simulink library "ddm"  (R2021b)
settings: Solver=VariableStepAuto  StartTime=0.0  StopTime=10.0  RelTol=1e-3
undefined symbols (not defined in the file or in its folder): ADDM_FrTMTqDev_X_Nm, ADDM_RrTMTqDev_X_Nm, ENUM_ADASACCSTA_ERROR, ENUM_ADASACCSTA_OFF, ENUM_ADASACCSTA_STANDBY, ENUM_ALLOWMOV_ALLOWREADY, ENUM_APS, ENUM_BRKSTA_ERROR, ENUM_BRKSTA_OFF, ENUM_BRKSTA_ON, ENUM_BRKSW_INVALID, ENUM_BRKSW_OFF, ENUM_BRKSW_ON, ENUM_CHGPREACTERRSTA_OBCPRE, ENUM_DCDCFAULTSTA_ANYFAULTLV1, ENUM_DCDCFAULTSTA_ANYFAULTLV2, ENUM_DRIVETRAIN_AWD, ENUM_DRIVETRAIN_FWD, ENUM_DRIVETRAIN_RWD, ENUM_EDUDRTSTA_NORMAL, ENUM_EPBSTA_APPLIED, ENUM_EPBSTA_RELEASED, ENUM_GEARACTUALPOSN_INVALID, ENUM_GEARACTUALPOSN_P, ENUM_HVBATTREADYPRE_READY, ENUM_MCUWARN_LV0, ENUM_MCUWARN_LV1, ENUM_MCUWARN_LV2, ENUM_MCUWARN_LV3, ENUM_MCUWARN_NOERROR, ENUM_OBCFAULTSTA_ANYFAULT, ENUM_PAS_R2F2, ENUM_PDFAULT_BATTPDFAIL, ENUM_PDFAULT_DCDCDISABLE, ENUM_PDFAULT_MCUDISABLE, ENUM_PDFAULT_MCUDISCHRG, ENUM_POWERSTA_OFF, ENUM_POWERSTA_ON, ENUM_POWERSTA_READY, ENUM_POWERSTA_STANDBY, ENUM_PRESSINDI_LOW, ENUM_PUFAULT_BATTUPFAIL, ENUM_PUFAULT_DCDCENABLEFAIL, ENUM_PUFAULT_PRECHRGCHKFAIL, ENUM_PUFAULT_SAFETYCHKFAIL, ENUM_PUSTATE_COMPLETED, ENUM_PWRSTASW_OFF, ENUM_PWRSTASW_OFFA, ENUM_PWRSTASW_OFFCHVCHRG, ENUM_PWRSTASW_OFFCLVCHRG, ENUM_PWRSTASW_ON, ENUM_PWRSTASW_ONHVCHRG, ENUM_PWRSTASW_READY, ENUM_PWRSTASW_STANDBY, ENUM_SHIFTCOMMAND_P, ENUM_SHIFTERERRSTA_PBUTTONFAILURE, ENUM_VEHMALFUNLV_2ND, ENUM_VEHMALFUNLV_3RD, ENUM_VEHMALFUNLV_4TH, ENUM_VEHMALFUNLV_NORMAL ... (+459)
libraries: hcu_lib x521, $bdroot x5, simulink x3
(part 22 of 25)

== system ddm/DDM/DDM/PMM/power up and power down/MCU active discharge fail ==
  note: Test Pass Criteria
  note: Test Detection Criteria
  note: Release Condition After Decision
  note: Diagnostics and Fault Handling
  task_time_s : Inport
  VPMM_PowerSta_enum : Inport  Port=2
  VPMM_PwrStaSW_enum : Inport  Port=3
  VPMM_PowerDownFault_enum : Inport  Port=4
  DTC_clear_request : Inport  Port=5
  VPMM_MCUDCBusMaxVolt_V : Inport  Port=6
  Constant : Constant  Value=ENUM_PDFAULT_MCUDISCHRG
  Constant1 : Constant  Value=FALSE
  Constant12 : Constant  Value=ENUM_PWRSTASW_OFF
  Constant13 : Constant  Value=FALSE
  Constant14 : Constant  Value=ZERO_INT
  Constant18 : Constant  Value=KPMM_MCUDischrgVolt_V
  Constant19 : Constant  Value=KDDM_MCUActDTC_cnt
  Constant2 : Constant  Value=TRUE
  Constant26 : Constant  Value=KDDM_MCUActDTC_cnt
  Constant29 : Constant  Value=FALSE
  Constant3 : Constant  Value=KDDM_PwrUpDnDiagnosisOffSW_flg
  Constant4 : Constant  Value=ENUM_POWERSTA_OFF
  Constant41 : Constant  Value=KDDM_MCUActDetTO_s
  Constant5 : Constant  Value=ENUM_PWRSTASW_OFF
  Constant6 : Constant  Value=TRUE
  Constant7 : Constant  Value=KDDM_MCUActPassTO_s
  Constant8 : Constant  Value=KDDM_MCUActPassTO_s
  Constant9 : Constant  Value=ENUM_POWERSTA_STANDBY
  DTC_Couter1 : hcu_lib/Basic_Blocks/DTC_Couter
  DTC_Info : hcu_lib/Basic_Blocks/DTC_Info
  Equal1 : RelationalOperator  Operator===  OutDataTypeStr=boolean  RndMeth=Simplest
  Equal11 : RelationalOperator  Operator=<=  OutDataTypeStr=boolean  RndMeth=Simplest
  Equal3 : RelationalOperator  Operator===  OutDataTypeStr=boolean  RndMeth=Simplest
  Equal5 : RelationalOperator  Operator=~=  OutDataTypeStr=boolean  RndMeth=Simplest
  Equal7 : RelationalOperator  Operator=~=  OutDataTypeStr=boolean  RndMeth=Simplest
  Equal8 : RelationalOperator  OutDataTypeStr=boolean  RndMeth=Simplest
  Equal9 : RelationalOperator  Operator===  OutDataTypeStr=boolean  RndMeth=Simplest
  Logical Operator13 : Logic  Operator=NOT  AllPortsSameDT=off  OutDataTypeStr=boolean
  Logical Operator14 : Logic  Operator=OR  Inputs=5  AllPortsSameDT=off  OutDataTypeStr=boolean
  Logical Operator16 : Logic  AllPortsSameDT=off  OutDataTypeStr=boolean
  Relational Operator1 : RelationalOperator  Operator=>  OutDataTypeStr=boolean  RndMeth=Simplest
  Switch{1..3,6} (4 alike) : Switch  Criteria=u2 ~= 0
  Terminator : Terminator
  Test Detection Criteria1 : hcu_lib/Basic_Blocks/Test Detection Criteria
  Timer2 : hcu_lib/Basic_Blocks/Timer
  Unit Delay1 : UnitDelay  SampleTime=-1  HasFrameUpgradeWarning=on
  VDDM_MCUActDTC_raw32 : Outport
  VDDM_MCUActDisFail_flg : Outport  Port=2
  VDDM_MCUActCFS_flg : Outport  Port=3
  wires:
  Switch1/1 -> VDDM_MCUActDisFail_flg/1  "VDDM_MCUActDisFail_flg"
  [VDDM_MCUActCFS_flg] -> Switch1/2, VDDM_MCUActCFS_flg/1
  Constant1/1 -> Switch1/3
  Constant2/1 -> Switch1/1
  [VDDM_MCUActPass_flg] -> Logical Operator14/3
  Constant18/1 -> Equal11/2
  Equal11/1 -> Logical Operator14/4
  [VPMM_MCUDCBusMaxVolt_V] -> Equal11/1
  Test Detection Criteria1/1 -> [VDDM_MCUActDet_flg]  "VDDM_MCUActDet_flg"
  Constant12/1 -> Equal7/2
  Relational Operator1/1 -> Terminator/1  "VDDM_MCUActDFS_flg"
  Constant7/1 -> Timer2/4
  Constant41/1 -> Test Detection Criteria1/4
  Logical Operator16/1 -> Logical Operator14/1
  [VPMM_PowerSta_enum] -> Unit Delay1/1
  [VPMM_PwrStaSW_enum] -> Equal7/1
  Timer2/1 -> Equal8/1
  DTC_Couter1/2 -> Relational Operator1/1  "VDDM_MCUActDTC_cnt"
  Constant4/1 -> Equal9/2
  [DTC_clear_request] -> Logical Operator14/2
  [VDDM_MCUActCFSRls_flg] -> DTC_Couter1/2
  [VPMM_PowerSta_enum] -> Equal3/1
  Unit Delay1/1 -> Equal9/1
  Constant9/1 -> Equal3/2
  Switch3/1 -> Switch6/3
  Logical Operator13/1 -> Timer2/1
  [VDDM_MCUActChk_flg] -> Switch3/1
  [task_time_s] -> Timer2/3
  Equal9/1 -> Logical Operator16/1
  Constant3/1 -> Logical Operator14/5
  Constant19/1 -> DTC_Couter1/3
  Switch2/1 -> Logical Operator13/1, Timer2/2
  Constant29/1 -> Switch6/1
  [task_time_s] -> Test Detection Criteria1/2
  Switch6/1 -> Test Detection Criteria1/1
  Constant5/1 -> Equal5/2
  Equal3/1 -> Logical Operator16/2
  Constant14/1 -> Relational Operator1/2
  Constant13/1 -> Switch3/3
  Constant8/1 -> Equal8/2
  Logical Operator14/1 -> [VDDM_MCUActCFSRls_flg]  "VDDM_MCUActCFSRls_flg"
  Constant26/1 -> Test Detection Criteria1/3
  [VDDM_MCUActDet_flg] -> DTC_Couter1/1
  Equal7/1 -> Switch3/2
  Constant6/1 -> Switch2/3
  [VDDM_MCUActCFSRls_flg] -> Switch6/2
  Equal8/1 -> [VDDM_MCUActPass_flg]  "VDDM_MCUActPass_flg"
  [VDDM_MCUActChk_flg] -> Switch2/1
  [VPMM_PwrStaSW_enum] -> Equal5/1
  Equal5/1 -> Switch2/2
  DTC_Couter1/1 -> [VDDM_MCUActCFS_flg]  "VDDM_MCUActCFS_flg"
  VPMM_PowerSta_enum/1 -> [VPMM_PowerSta_enum]
  VPMM_PwrStaSW_enum/1 -> [VPMM_PwrStaSW_enum]
  task_time_s/1 -> [task_time_s]
  DTC_clear_request/1 -> [DTC_clear_request]
  Constant/1 -> Equal1/2
  VPMM_PowerDownFault_enum/1 -> Equal1/1
  Equal1/1 -> [VDDM_MCUActChk_flg]
  DTC_Info/1 -> VDDM_MCUActDTC_raw32/1  "VDDM_MCUActDTC_raw32"
  [VDDM_MCUActPass_flg] -> DTC_Info/2
  [VDDM_MCUActCFS_flg] -> DTC_Info/3
  [VDDM_MCUActDet_flg] -> DTC_Info/1
  [DTC_clear_request] -> DTC_Info/4
  VPMM_MCUDCBusMaxVolt_V/1 -> [VPMM_MCUDCBusMaxVolt_V]

== system ddm/DDM/DDM/PMM/power up and power down/MCU disable fail ==
  note: Test Detection Criteria
  note: Test Pass Criteria
  note: Diagnostics and Fault Handling
  note: Release Condition After Decision
  task_time_s : Inport
  VPMM_PowerSta_enum : Inport  Port=2
  VPMM_PwrStaSW_enum : Inport  Port=3
  VPMM_PowerDownFault_enum : Inport  Port=4
  DTC_clear_request : Inport  Port=5
  Constant : Constant  Value=ENUM_PDFAULT_MCUDISABLE
  Constant1 : Constant  Value=KDDM_PwrUpDnDiagnosisOffSW_flg
  Constant12 : Constant  Value=ENUM_PWRSTASW_OFF
  Constant13 : Constant  Value=FALSE
  Constant14 : Constant  Value=ZERO_INT
  Constant18 : Constant  Value=KDDM_MCUDisDTC_cnt
  Constant2 : Constant  Value=ENUM_PWRSTASW_OFF
  Constant23 : Constant  Value=TRUE
  Constant26 : Constant  Value=KDDM_MCUDisDTC_cnt
  Constant29 : Constant  Value=FALSE
  Constant3 : Constant  Value=ENUM_POWERSTA_OFF
  Constant4 : Constant  Value=KDDM_MCUDisPassTO_s
  Constant41 : Constant  Value=KDDM_MCUDisDetTO_s
  Constant8 : Constant  Value=ENUM_POWERSTA_STANDBY
  Constant9 : Constant  Value=KDDM_MCUDisPassTO_s
  DTC_Couter1 : hcu_lib/Basic_Blocks/DTC_Couter
  DTC_Info : hcu_lib/Basic_Blocks/DTC_Info
  Equal1 : RelationalOperator  Operator===  OutDataTypeStr=boolean  RndMeth=Simplest
  Equal10 : RelationalOperator  Operator===  OutDataTypeStr=boolean  RndMeth=Simplest
  Equal2 : RelationalOperator  Operator=~=  OutDataTypeStr=boolean  RndMeth=Simplest
  Equal5 : RelationalOperator  Operator=~=  OutDataTypeStr=boolean  RndMeth=Simplest
  Equal8 : RelationalOperator  OutDataTypeStr=boolean  RndMeth=Simplest
  Equal9 : RelationalOperator  Operator===  OutDataTypeStr=boolean  RndMeth=Simplest
  Logical Operator13 : Logic  Operator=NOT  AllPortsSameDT=off  OutDataTypeStr=boolean
  Logical Operator14 : Logic  Operator=OR  Inputs=4  AllPortsSameDT=off  OutDataTypeStr=boolean
  Logical Operator16 : Logic  AllPortsSameDT=off  OutDataTypeStr=boolean
  Relational Operator1 : RelationalOperator  Operator=>  OutDataTypeStr=boolean  RndMeth=Simplest
  Switch1 : Switch  Criteria=u2 ~= 0
  Switch3 : Switch  Criteria=u2 ~= 0
  Switch6 : Switch  Criteria=u2 ~= 0
  Terminator : Terminator
  Test Detection Criteria1 : hcu_lib/Basic_Blocks/Test Detection Criteria
  Timer2 : hcu_lib/Basic_Blocks/Timer
  Unit Delay1 : UnitDelay  SampleTime=-1  HasFrameUpgradeWarning=on
  VDDM_MCUDisDTC_raw32 : Outport
  VDDM_MCUDisCFS_flg : Outport  Port=2
  wires:
  [VDDM_MCUDisCFS_flg] -> VDDM_MCUDisCFS_flg/1
  Constant23/1 -> Switch1/3
  [VDDM_MCUDisChk_flg] -> Switch1/1
  Equal2/1 -> Switch1/2
  Constant2/1 -> Equal2/2
  [VPMM_PwrStaSW_enum] -> Equal2/1
  DTC_Couter1/1 -> [VDDM_MCUDisCFS_flg]  "VDDM_MCUDisCFS_flg"
  [VPMM_PwrStaSW_enum] -> Equal5/1
  Equal8/1 -> [VDDM_MCUDisPass_flg]  "VDDM_MCUDisPass_flg"
  [task_time_s] -> Test Detection Criteria1/2
  Constant26/1 -> Test Detection Criteria1/3
  Unit Delay1/1 -> Equal9/1
  [VDDM_MCUDisChk_flg] -> Switch3/1
  Test Detection Criteria1/1 -> [VDDM_MCUDisDet_flg]  "VDDM_MCUDisDet_flg"
  Equal10/1 -> Logical Operator16/2
  DTC_Couter1/2 -> Relational Operator1/1  "VDDM_MCUDisDTC_cnt"
  Switch6/1 -> Test Detection Criteria1/1
  Constant4/1 -> Timer2/4
  Switch1/1 -> Logical Operator13/1, Timer2/2
  Logical Operator14/1 -> [VDDM_MCUDisCFSRls_flg]  "VDDM_MCUDisCFSRls_flg"
  Switch3/1 -> Switch6/3
  Constant13/1 -> Switch3/3
  Constant14/1 -> Relational Operator1/2
  [VDDM_MCUDisPass_flg] -> Logical Operator14/3
  [DTC_clear_request] -> Logical Operator14/2
  Constant29/1 -> Switch6/1
  Equal5/1 -> Switch3/2
  Constant9/1 -> Equal8/2
  [VDDM_MCUDisCFSRls_flg] -> DTC_Couter1/2
  Constant41/1 -> Test Detection Criteria1/4
  Logical Operator16/1 -> Logical Operator14/1
  Constant12/1 -> Equal5/2
  Logical Operator13/1 -> Timer2/1
  Equal9/1 -> Logical Operator16/1
  Timer2/1 -> Equal8/1
  Constant18/1 -> DTC_Couter1/3
  Constant1/1 -> Logical Operator14/4
  [VPMM_PowerSta_enum] -> Unit Delay1/1
  [VPMM_PowerSta_enum] -> Equal10/1
  Constant3/1 -> Equal9/2
  Constant8/1 -> Equal10/2
  [task_time_s] -> Timer2/3
  [VDDM_MCUDisDet_flg] -> DTC_Couter1/1
  Relational Operator1/1 -> Terminator/1  "VDDM_MCUDisDFS_flg"
  [VDDM_MCUDisCFSRls_flg] -> Switch6/2
  task_time_s/1 -> [task_time_s]
  VPMM_PwrStaSW_enum/1 -> [VPMM_PwrStaSW_enum]
  VPMM_PowerSta_enum/1 -> [VPMM_PowerSta_enum]
  Constant/1 -> Equal1/2
  VPMM_PowerDownFault_enum/1 -> Equal1/1
  DTC_clear_request/1 -> [DTC_clear_request]
  Equal1/1 -> [VDDM_MCUDisChk_flg]
  DTC_Info/1 -> VDDM_MCUDisDTC_raw32/1  "VDDM_MCUDisDTC_raw32"
  [VDDM_MCUDisPass_flg] -> DTC_Info/2
  [VDDM_MCUDisCFS_flg] -> DTC_Info/3
  [VDDM_MCUDisDet_flg] -> DTC_Info/1
  [DTC_clear_request] -> DTC_Info/4

== system ddm/DDM/DDM/PMM/power up and power down/MCU ready for precharge fail ==
  note: Diagnostics and Fault Handling
  note: Test Detection Criteria
  note: Test Pass Criteria
  note: Release Condition After Decision
  task_time_s : Inport
  VPMM_PowerSta_enum : Inport  Port=2
  VPMM_PwrStaSW_enum : Inport  Port=3
  VPMM_MCUReady4Pre_flg : Inport  Port=4
  VPMM_PowerUpFault_enum : Inport  Port=5
  DTC_clear_request : Inport  Port=6
  VPMM_PowerUpState_enum : Inport  Port=7
  Constant : Constant  Value=ENUM_PUFAULT_PRECHRGCHKFAIL
  Constant12 : Constant  Value=ENUM_PWRSTASW_OFF
  Constant13 : Constant  Value=FALSE
  Constant14 : Constant  Value=ZERO_INT
  Constant17 : Constant  Value=KDDM_PwrUpDnDiagnosisOffSW_flg
  Constant18 : Constant  Value=KDDM_MCU4PrePassTO_s
  Constant22 : Constant  Value=ENUM_POWERSTA_OFF
  Constant28 : Constant  Value=KDDM_MCU4PrePassTO_s
  Constant29 : Constant  Value=FALSE
  Constant3 : Constant  Value=KDDM_MCU4PreDTC_cnt
  Constant4 : Constant  Value=FALSE
  Constant41 : Constant  Value=KDDM_MCU4PreDetTO_s
  Constant5 : Constant  Value=ENUM_PUSTATE_COMPLETED
  Constant6 : Constant  Value=TRUE
  Constant7 : Constant  Value=ENUM_POWERSTA_STANDBY
  Constant9 : Constant  Value=KDDM_MCU4PreDTC_cnt
  DTC_Couter1 : hcu_lib/Basic_Blocks/DTC_Couter
  DTC_Info : hcu_lib/Basic_Blocks/DTC_Info
  Equal{1,3,8..9} (4 alike) : RelationalOperator  Operator===  OutDataTypeStr=boolean  RndMeth=Simplest
  Equal4 : RelationalOperator  Operator=~=  OutDataTypeStr=boolean  RndMeth=Simplest
  Equal7 : RelationalOperator  OutDataTypeStr=boolean  RndMeth=Simplest
  Logical Operator13 : Logic  Operator=NOT  AllPortsSameDT=off  OutDataTypeStr=boolean
  Logical Operator14 : Logic  Operator=OR  Inputs=4  AllPortsSameDT=off  OutDataTypeStr=boolean
  Logical Operator16 : Logic  AllPortsSameDT=off  OutDataTypeStr=boolean
  Logical Operator4 : Logic  AllPortsSameDT=off  OutDataTypeStr=boolean
  Logical Operator5 : Logic  Operator=NOT  AllPortsSameDT=off  OutDataTypeStr=boolean
  Relational Operator1 : RelationalOperator  Operator=>  OutDataTypeStr=boolean  RndMeth=Simplest
  Switch1 : Switch  Criteria=u2 ~= 0
  Switch3 : Switch  Criteria=u2 ~= 0
  Switch6 : Switch  Criteria=u2 ~= 0
  Terminator : Terminator
  Test Detection Criteria1 : hcu_lib/Basic_Blocks/Test Detection Criteria
  Timer2 : hcu_lib/Basic_Blocks/Timer
  Unit Delay1 : UnitDelay  SampleTime=-1  HasFrameUpgradeWarning=on
  VDDM_MCU4PreDTC_raw32 : Outport
  VDDM_MCU4PreCFS_flg : Outport  Port=2
  wires:
  [VDDM_MCU4PreCFS_flg] -> VDDM_MCU4PreCFS_flg/1
  Constant9/1 -> Test Detection Criteria1/3
  [VDDM_MCU4PreCFSRls_flg] -> DTC_Couter1/2
  Test Detection Criteria1/1 -> [VDDM_MCU4PreDet_flg]  "VDDM_MCU4PreDet_flg"
  Logical Operator14/1 -> [VDDM_MCU4PreCFSRls_flg]  "VDDM_MCU4PreCFSRls_flg"
  Constant4/1 -> Switch1/1
  Switch1/1 -> Logical Operator13/1, Timer2/2
  [DTC_clear_request] -> Logical Operator14/2
  [VPMM_PowerSta_enum] -> Unit Delay1/1
  Constant14/1 -> Relational Operator1/2
  Equal3/1 -> Switch1/2
  Equal4/1 -> Switch3/2
  Switch3/1 -> Switch6/3
  [VPMM_PowerSta_enum] -> Equal9/1
  [VDDM_MCU4PrePass_flg] -> Logical Operator14/3
  Constant7/1 -> Equal9/2
  Constant5/1 -> Equal3/2
  Constant29/1 -> Switch6/1
  Unit Delay1/1 -> Equal8/1
  Constant12/1 -> Equal4/2
  Constant17/1 -> Logical Operator14/4
  [task_time_s] -> Test Detection Criteria1/2
  [VDDM_MCU4PreCFSRls_flg] -> Switch6/2
  [VDDM_MCU4PreDet_flg] -> DTC_Couter1/1
  Constant22/1 -> Equal8/2
  Constant13/1 -> Switch3/3
  Constant3/1 -> DTC_Couter1/3
  Switch6/1 -> Test Detection Criteria1/1
  Equal9/1 -> Logical Operator16/2
  Logical Operator13/1 -> Timer2/1
  DTC_Couter1/2 -> Relational Operator1/1  "VDDM_MCU4PreDTC_cnt"
  Constant6/1 -> Switch1/3
  Constant41/1 -> Test Detection Criteria1/4
  [task_time_s] -> Timer2/3
  [VPMM_PowerUpState_enum] -> Equal3/1
  Equal8/1 -> Logical Operator16/1
  Timer2/1 -> Equal7/1
  Logical Operator16/1 -> Logical Operator14/1
  Equal7/1 -> [VDDM_MCU4PrePass_flg]  "VDDM_MCU4PrePass_flg"
  [VPMM_PwrStaSW_enum] -> Equal4/1
  [VDDM_MCU4PreChk_flg] -> Switch3/1
  Relational Operator1/1 -> Terminator/1  "VDDM_MCU4PreDFS_flg"
  Constant28/1 -> Equal7/2
  DTC_Couter1/1 -> [VDDM_MCU4PreCFS_flg]  "VDDM_MCU4PreCFS_flg"
  Constant18/1 -> Timer2/4
  task_time_s/1 -> [task_time_s]
  VPMM_PwrStaSW_enum/1 -> [VPMM_PwrStaSW_enum]
  VPMM_PowerSta_enum/1 -> [VPMM_PowerSta_enum]
  DTC_clear_request/1 -> [DTC_clear_request]
  Constant/1 -> Equal1/2
  VPMM_PowerUpFault_enum/1 -> Equal1/1
  Logical Operator5/1 -> Logical Operator4/1
  Equal1/1 -> Logical Operator4/2
  Logical Operator4/1 -> [VDDM_MCU4PreChk_flg]
  VPMM_MCUReady4Pre_flg/1 -> Logical Operator5/1
  [VDDM_MCU4PrePass_flg] -> DTC_Info/2
  DTC_Info/1 -> VDDM_MCU4PreDTC_raw32/1  "VDDM_MCU4PreDTC_raw32"
  [VDDM_MCU4PreCFS_flg] -> DTC_Info/3
  [VDDM_MCU4PreDet_flg] -> DTC_Info/1
  [DTC_clear_request] -> DTC_Info/4
  VPMM_PowerUpState_enum/1 -> [VPMM_PowerUpState_enum]

== system ddm/DDM/DDM/PMM/power up and power down/Mid level system safety check fail ==
  note: Release Condition After Decision
  note: Diagnostics and Fault Handling
  note: Test Detection Criteria
  note: Test Pass Criteria
  task_time_s : Inport
  VPMM_PowerSta_enum : Inport  Port=2
  VPMM_PwrStaSW_enum : Inport  Port=3
  VDDM_MidLvSaChkChk_flg : Inport  Port=4
  VPMM_PowerUpFault_enum : Inport  Port=5
  DTC_clear_request : Inport  Port=6
  VPMM_PowerUpState_enum : Inport  Port=7
  Constant : Constant  Value=ENUM_PUFAULT_SAFETYCHKFAIL
  Constant12 : Constant  Value=ENUM_PWRSTASW_OFF
  Constant13 : Constant  Value=FALSE
  Constant14 : Constant  Value=ZERO_INT
  Constant17 : Constant  Value=KDDM_PwrUpDnDiagnosisOffSW_flg
  Constant18 : Constant  Value=KDDM_MidLvSaChkDTC_cnt
  Constant22 : Constant  Value=ENUM_POWERSTA_OFF
  Constant28 : Constant  Value=KDDM_MidLvSaChkPassTO_s
  Constant29 : Constant  Value=FALSE
  Constant3 : Constant  Value=KDDM_MidLvSaChkDTC_cnt
  Constant30 : Constant  Value=KDDM_MidLvSaChkPassTO_s
  Constant4 : Constant  Value=FALSE
  Constant41 : Constant  Value=KDDM_MidLvSaChkDetTO_s
  Constant5 : Constant  Value=ENUM_PUSTATE_COMPLETED
  Constant6 : Constant  Value=TRUE
  Constant7 : Constant  Value=ENUM_POWERSTA_STANDBY
  DTC_Couter1 : hcu_lib/Basic_Blocks/DTC_Couter
  DTC_Info : hcu_lib/Basic_Blocks/DTC_Info
  Equal{1,3,8..9} (4 alike) : RelationalOperator  Operator===  OutDataTypeStr=boolean  RndMeth=Simplest
  Equal4 : RelationalOperator  Operator=~=  OutDataTypeStr=boolean  RndMeth=Simplest
  Equal7 : RelationalOperator  OutDataTypeStr=boolean  RndMeth=Simplest
  Logical Operator13 : Logic  Operator=NOT  AllPortsSameDT=off  OutDataTypeStr=boolean
  Logical Operator14 : Logic  Operator=OR  Inputs=4  AllPortsSameDT=off  OutDataTypeStr=boolean
  Logical Operator16 : Logic  AllPortsSameDT=off  OutDataTypeStr=boolean
  Logical Operator4 : Logic  Operator=NOT  AllPortsSameDT=off  OutDataTypeStr=boolean
  Logical Operator5 : Logic  AllPortsSameDT=off  OutDataTypeStr=boolean
  Relational Operator1 : RelationalOperator  Operator=>  OutDataTypeStr=boolean  RndMeth=Simplest
  Switch1 : Switch  Criteria=u2 ~= 0
  Switch3 : Switch  Criteria=u2 ~= 0
  Switch6 : Switch  Criteria=u2 ~= 0
  Terminator : Terminator
  Test Detection Criteria1 : hcu_lib/Basic_Blocks/Test Detection Criteria
  Timer2 : hcu_lib/Basic_Blocks/Timer
  Unit Delay1 : UnitDelay  SampleTime=-1  HasFrameUpgradeWarning=on
  VDDM_MidLvSaChkDTC_raw32 : Outport
  VDDM_MidLvSaChkCFS_flg : Outport  Port=2
  wires:
  [VDDM_MidLvSaChkCFS_flg] -> VDDM_MidLvSaChkCFS_flg/1
  Equal4/1 -> Switch3/2
  Relational Operator1/1 -> Terminator/1  "VDDM_MidLvSaChkDFS_flg"
  [DTC_clear_request] -> Logical Operator14/2
  Constant29/1 -> Switch6/1
  Logical Operator14/1 -> [VDDM_MidLvSaChkCFSRls_flg]  "VDDM_MidLvSaChkCFSRls_flg"
  [VDDM_MidLvSaChkPass_flg] -> Logical Operator14/3
  Constant6/1 -> Switch1/3
  [task_time_s] -> Test Detection Criteria1/2
  Constant14/1 -> Relational Operator1/2
  Constant13/1 -> Switch3/3
  DTC_Couter1/1 -> [VDDM_MidLvSaChkCFS_flg]  "VDDM_MidLvSaChkCFS_flg"
  Equal7/1 -> [VDDM_MidLvSaChkPass_flg]  "VDDM_MidLvSaChkPass_flg"
  Switch1/1 -> Logical Operator13/1, Timer2/2
  Switch3/1 -> Switch6/3
  Constant28/1 -> Timer2/4
  Constant5/1 -> Equal3/2
  [VPMM_PwrStaSW_enum] -> Equal4/1
  Equal9/1 -> Logical Operator16/2
  Constant30/1 -> Equal7/2
  Constant3/1 -> Test Detection Criteria1/3
  DTC_Couter1/2 -> Relational Operator1/1  "VDDM_MidLvSaChkDTC_cnt"
  Constant4/1 -> Switch1/1
  [VPMM_PowerUpState_enum] -> Equal3/1
  Unit Delay1/1 -> Equal8/1
  Constant7/1 -> Equal9/2
  [task_time_s] -> Timer2/3
  Constant22/1 -> Equal8/2
  [VPMM_PowerSta_enum] -> Equal9/1
  Constant17/1 -> Logical Operator14/4
  Switch6/1 -> Test Detection Criteria1/1
  [VPMM_PowerSta_enum] -> Unit Delay1/1
  Logical Operator13/1 -> Timer2/1
  [VDDM_MidLvSaChkChk_flg] -> Switch3/1
  Timer2/1 -> Equal7/1
  Constant12/1 -> Equal4/2
  Equal8/1 -> Logical Operator16/1
  Equal3/1 -> Switch1/2
  Constant41/1 -> Test Detection Criteria1/4
  Logical Operator16/1 -> Logical Operator14/1
  Test Detection Criteria1/1 -> [VDDM_MidLvSaChkDet_flg]  "VDDM_MidLvSaChkDet_flg"
  [VDDM_MidLvSaChkCFSRls_flg] -> DTC_Couter1/2
  [VDDM_MidLvSaChkDet_flg] -> DTC_Couter1/1
  [VDDM_MidLvSaChkCFSRls_flg] -> Switch6/2
  Constant18/1 -> DTC_Couter1/3
  VPMM_PowerSta_enum/1 -> [VPMM_PowerSta_enum]
  VPMM_PwrStaSW_enum/1 -> [VPMM_PwrStaSW_enum]
  task_time_s/1 -> [task_time_s]
  Constant/1 -> Equal1/2
  Equal1/1 -> Logical Operator5/2
  Logical Operator4/1 -> Logical Operator5/1
  VPMM_PowerUpFault_enum/1 -> Equal1/1
  Logical Operator5/1 -> [VDDM_MidLvSaChkChk_flg]
  VDDM_MidLvSaChkChk_flg/1 -> Logical Operator4/1
  DTC_clear_request/1 -> [DTC_clear_request]
  DTC_Info/1 -> VDDM_MidLvSaChkDTC_raw32/1  "VDDM_MidLvSaChkDTC_raw32"
  [VDDM_MidLvSaChkPass_flg] -> DTC_Info/2
  [VDDM_MidLvSaChkCFS_flg] -> DTC_Info/3
  [VDDM_MidLvSaChkDet_flg] -> DTC_Info/1
  [DTC_clear_request] -> DTC_Info/4
  VPMM_PowerUpState_enum/1 -> [VPMM_PowerUpState_enum]

== system ddm/DDM/DDM/PMM/power up and power down/OBC ready for precharge fail ==
  note: Release Condition After Decision
  note: Test Detection Criteria
  note: Diagnostics and Fault Handling
  note: Test Pass Criteria
  task_time_s : Inport
  VPMM_PowerSta_enum : Inport  Port=2
  VPMM_PwrStaSW_enum : Inport  Port=3
  VPMM_HVChrgPreActionErrSta_enum : Inport  Port=4
  DTC_clear_request : Inport  Port=5
  Constant12 : Constant  Value=ENUM_PWRSTASW_OFFCLVCHRG
  Constant13 : Constant  Value=ENUM_PWRSTASW_ONHVCHRG
  Constant14 : Constant  Value=ZERO_INT
  Constant22 : Constant  Value=ENUM_PWRSTASW_ON
  Constant28 : Constant  Value=FALSE
  Constant29 : Constant  Value=ENUM_PWRSTASW_OFFCHVCHRG
  Constant3 : Constant  Value=ENUM_CHGPREACTERRSTA_OBCPRE
  Constant30 : Constant  Value=KDDM_OBC4PreDetTO_s
  Constant31 : Constant  Value=FALSE
  Constant32 : Constant  Value=ENUM_POWERSTA_OFF
  Constant33 : Constant  Value=KDDM_OBC4PreDTC_cnt
  Constant34 : Constant  Value=ENUM_POWERSTA_STANDBY
  Constant35 : Constant  Value=ENUM_PWRSTASW_OFFCLVCHRG
  Constant36 : Constant  Value=TRUE
  Constant37 : Constant  Value=ENUM_PWRSTASW_ONHVCHRG
  Constant39 : Constant  Value=ENUM_PWRSTASW_ON
  Constant41 : Constant  Value=ENUM_PWRSTASW_OFFCHVCHRG
  Constant42 : Constant  Value=KDDM_OBC4PrePassTO_s
  Constant45 : Constant  Value=KDDM_OBC4PrePassTO_s
  Constant46 : Constant  Value=KDDM_OBC4PreDTC_cnt
  Constant9 : Constant  Value=KDDM_PwrUpDnDiagnosisOffSW_flg
  DTC_Couter1 : hcu_lib/Basic_Blocks/DTC_Couter
  DTC_Info : hcu_lib/Basic_Blocks/DTC_Info
  Equal{10..12,14..20,24} (11 alike) : RelationalOperator  Operator===  OutDataTypeStr=boolean  RndMeth=Simplest
  Equal13 : RelationalOperator  OutDataTypeStr=boolean  RndMeth=Simplest
  Logical Operator10 : Logic  Operator=OR  Inputs=4  AllPortsSameDT=off  OutDataTypeStr=boolean
  Logical Operator13 : Logic  Operator=NOT  AllPortsSameDT=off  OutDataTypeStr=boolean
  Logical Operator14 : Logic  Operator=OR  Inputs=4  AllPortsSameDT=off  OutDataTypeStr=boolean
  Logical Operator16 : Logic  AllPortsSameDT=off  OutDataTypeStr=boolean
  Logical Operator9 : Logic  Operator=OR  Inputs=4  AllPortsSameDT=off  OutDataTypeStr=boolean
  Relational Operator1 : RelationalOperator  Operator=>  OutDataTypeStr=boolean  RndMeth=Simplest
  Switch3 : Switch  Criteria=u2 ~= 0
  Switch6 : Switch  Criteria=u2 ~= 0
  Switch7 : Switch  Criteria=u2 ~= 0
  Terminator : Terminator
  Test Detection Criteria1 : hcu_lib/Basic_Blocks/Test Detection Criteria
  Timer2 : hcu_lib/Basic_Blocks/Timer
  Unit Delay1 : UnitDelay  SampleTime=-1  HasFrameUpgradeWarning=on
  VDDM_OBC4PreDTC_raw32 : Outport
  VDDM_OBC4PreCFS_flg : Outport  Port=2
  wires:
  [VDDM_OBC4PreCFS_flg] -> VDDM_OBC4PreCFS_flg/1
  Constant39/1 -> Equal17/2
  [VPMM_PwrStaSW_enum] -> Equal17/1
  Equal19/1 -> Logical Operator10/1
  [VPMM_PwrStaSW_enum] -> Equal19/1
  [VPMM_PwrStaSW_enum] -> Equal20/1
  Constant41/1 -> Equal19/2
  Equal20/1 -> Logical Operator10/4
  Constant37/1 -> Equal20/2
  Constant36/1 -> Switch6/3
  [VDDM_OBC4PreChk_flg] -> Switch6/1
  Equal18/1 -> Logical Operator10/3
  [VPMM_PwrStaSW_enum] -> Equal18/1
  Constant35/1 -> Equal18/2
  Equal17/1 -> Logical Operator10/2
  Logical Operator10/1 -> Switch6/2
  [VPMM_PwrStaSW_enum] -> Equal15/1
  Equal16/1 -> Logical Operator9/4
  Equal15/1 -> Logical Operator9/1
  [VDDM_OBC4PreChk_flg] -> Switch3/1
  Constant28/1 -> Switch3/3
  [VPMM_PwrStaSW_enum] -> Equal11/1
  [VPMM_PwrStaSW_enum] -> Equal12/1
  Constant12/1 -> Equal12/2
  Logical Operator9/1 -> Switch3/2
  Constant29/1 -> Equal15/2
  Equal11/1 -> Logical Operator9/2
  Equal12/1 -> Logical Operator9/3
  Constant13/1 -> Equal16/2
  Constant22/1 -> Equal11/2
  [VPMM_PwrStaSW_enum] -> Equal16/1
  Constant46/1 -> DTC_Couter1/3
  Timer2/1 -> Equal13/1
  [VDDM_OBC4PrePass_flg] -> Logical Operator14/3
  [VDDM_OBC4PreCFSRls_flg] -> Switch7/2
  Switch7/1 -> Test Detection Criteria1/1
  Switch6/1 -> Logical Operator13/1, Timer2/2
  Equal14/1 -> Logical Operator16/1
  Constant33/1 -> Test Detection Criteria1/3
  Equal13/1 -> [VDDM_OBC4PrePass_flg]  "VDDM_OBC4PrePass_flg"
  Constant30/1 -> Test Detection Criteria1/4
  DTC_Couter1/2 -> Relational Operator1/1  "VDDM_OBC4PreDTC_cnt"
  Equal10/1 -> Logical Operator16/2
  [VDDM_OBC4PreCFSRls_flg] -> DTC_Couter1/2
  Unit Delay1/1 -> Equal14/1
  Test Detection Criteria1/1 -> [VDDM_OBC4PreDet_flg]  "VDDM_OBC4PreDet_flg"
  [task_time_s] -> Test Detection Criteria1/2
  [VDDM_OBC4PreDet_flg] -> DTC_Couter1/1
  [task_time_s] -> Timer2/3
  [VPMM_PowerSta_enum] -> Unit Delay1/1
  Constant9/1 -> Logical Operator14/4
  [VPMM_PowerSta_enum] -> Equal10/1
  Constant34/1 -> Equal10/2
  Constant32/1 -> Equal14/2
  Logical Operator13/1 -> Timer2/1
  Logical Operator16/1 -> Logical Operator14/1
  Logical Operator14/1 -> [VDDM_OBC4PreCFSRls_flg]  "VDDM_OBC4PreCFSRls_flg"
  Relational Operator1/1 -> Terminator/1  "VDDM_OBC4PreDFS_flg"
  Switch3/1 -> Switch7/3
  Constant31/1 -> Switch7/1
  DTC_Couter1/1 -> [VDDM_OBC4PreCFS_flg]  "VDDM_OBC4PreCFS_flg"
  [DTC_clear_request] -> Logical Operator14/2
  Constant14/1 -> Relational Operator1/2
  Constant42/1 -> Timer2/4
  Constant45/1 -> Equal13/2
  task_time_s/1 -> [task_time_s]
  VPMM_PwrStaSW_enum/1 -> [VPMM_PwrStaSW_enum]
  VPMM_PowerSta_enum/1 -> [VPMM_PowerSta_enum]
  Constant3/1 -> Equal24/2
  VPMM_HVChrgPreActionErrSta_enum/1 -> Equal24/1
  Equal24/1 -> [VDDM_OBC4PreChk_flg]  "VDDM_OBC4PreChk_flg"
  DTC_clear_request/1 -> [DTC_clear_request]
  DTC_Info/1 -> VDDM_OBC4PreDTC_raw32/1  "VDDM_OBC4PreDTC_raw32"
  [VDDM_OBC4PrePass_flg] -> DTC_Info/2
  [VDDM_OBC4PreCFS_flg] -> DTC_Info/3
  [VDDM_OBC4PreDet_flg] -> DTC_Info/1
  [DTC_clear_request] -> DTC_Info/4

== system ddm/DDM/DDM/TPM/LFBatwarn/SR_Latch1 ==
  set : Inport
  reset : Inport  Port=2
  Logical Operator : Logic  AllPortsSameDT=off  OutDataTypeStr=boolean
  Logical Operator1 : Logic  Operator=NOT  AllPortsSameDT=off  OutDataTypeStr=boolean
  Switch1 : Switch  Criteria=u2 ~= 0  Threshold=0.5
      settings: AttributesFormatString=<Criteria=%<Criteria>>
  Switch2 : Switch  Criteria=u2 ~= 0  Threshold=0.5
      settings: AttributesFormatString=<Criteria=%<Criteria>>
  Unit Delay : UnitDelay  SampleTime=-1  HasFrameUpgradeWarning=on
  latched : Outport
  wires:
  Switch1/1 -> Unit Delay/1, latched/1
  set/1 -> Switch1/1, Logical Operator/1
  reset/1 -> Switch2/2, Logical Operator1/1
  Unit Delay/1 -> Switch2/3
  Switch2/1 -> Switch1/3
  Logical Operator/1 -> Switch1/2
  Logical Operator1/1 -> Logical Operator/2, Switch2/1

== system ddm/DDM/DDM/TPM/LFPressureLow/SR_Latch1 ==
  set : Inport
  reset : Inport  Port=2
  Logical Operator : Logic  AllPortsSameDT=off  OutDataTypeStr=boolean
  Logical Operator1 : Logic  Operator=NOT  AllPortsSameDT=off  OutDataTypeStr=boolean
  Switch1 : Switch  Criteria=u2 ~= 0  Threshold=0.5
      settings: AttributesFormatString=<Criteria=%<Criteria>>
  Switch2 : Switch  Criteria=u2 ~= 0  Threshold=0.5
      settings: AttributesFormatString=<Criteria=%<Criteria>>
  Unit Delay : UnitDelay  SampleTime=-1  HasFrameUpgradeWarning=on
  latched : Outport
  wires:
  Switch1/1 -> Unit Delay/1, latched/1
  set/1 -> Switch1/1, Logical Operator/1
  reset/1 -> Switch2/2, Logical Operator1/1
  Unit Delay/1 -> Switch2/3
  Switch2/1 -> Switch1/3
  Logical Operator/1 -> Switch1/2
  Logical Operator1/1 -> Logical Operator/2, Switch2/1

== system ddm/DDM/DDM/TPM/LFSensorfail/SR_Latch1 ==
  set : Inport
  reset : Inport  Port=2
  Logical Operator : Logic  AllPortsSameDT=off  OutDataTypeStr=boolean
  Logical Operator1 : Logic  Operator=NOT  AllPortsSameDT=off  OutDataTypeStr=boolean
  Switch1 : Switch  Criteria=u2 ~= 0  Threshold=0.5
      settings: AttributesFormatString=<Criteria=%<Criteria>>
  Switch2 : Switch  Criteria=u2 ~= 0  Threshold=0.5
      settings: AttributesFormatString=<Criteria=%<Criteria>>
  Unit Delay : UnitDelay  SampleTime=-1  HasFrameUpgradeWarning=on
  latched : Outport
  wires:
  Switch1/1 -> Unit Delay/1, latched/1
  set/1 -> Switch1/1, Logical Operator/1
  reset/1 -> Switch2/2, Logical Operator1/1
  Unit Delay/1 -> Switch2/3
  Switch2/1 -> Switch1/3
  Logical Operator/1 -> Switch1/2
  Logical Operator1/1 -> Logical Operator/2, Switch2/1

== system ddm/DDM/DDM/TPM/LFWheelTmpHigh/SR_Latch1 ==
  set : Inport
  reset : Inport  Port=2
  Logical Operator : Logic  AllPortsSameDT=off  OutDataTypeStr=boolean
  Logical Operator1 : Logic  Operator=NOT  AllPortsSameDT=off  OutDataTypeStr=boolean
  Switch1 : Switch  Criteria=u2 ~= 0  Threshold=0.5
      settings: AttributesFormatString=<Criteria=%<Criteria>>
  Switch2 : Switch  Criteria=u2 ~= 0  Threshold=0.5
      settings: AttributesFormatString=<Criteria=%<Criteria>>
  Unit Delay : UnitDelay  SampleTime=-1  HasFrameUpgradeWarning=on
  latched : Outport
  wires:
  Switch1/1 -> Unit Delay/1, latched/1
  set/1 -> Switch1/1, Logical Operator/1
  reset/1 -> Switch2/2, Logical Operator1/1
  Unit Delay/1 -> Switch2/3
  Switch2/1 -> Switch1/3
  Logical Operator/1 -> Switch1/2
  Logical Operator1/1 -> Logical Operator/2, Switch2/1

== system ddm/DDM/DDM/TPM/LRBatwarn/SR_Latch1 ==
  set : Inport
  reset : Inport  Port=2
  Logical Operator : Logic  AllPortsSameDT=off  OutDataTypeStr=boolean
  Logical Operator1 : Logic  Operator=NOT  AllPortsSameDT=off  OutDataTypeStr=boolean
  Switch1 : Switch  Criteria=u2 ~= 0  Threshold=0.5
      settings: AttributesFormatString=<Criteria=%<Criteria>>
  Switch2 : Switch  Criteria=u2 ~= 0  Threshold=0.5
      settings: AttributesFormatString=<Criteria=%<Criteria>>
  Unit Delay : UnitDelay  SampleTime=-1  HasFrameUpgradeWarning=on
  latched : Outport
  wires:
  Switch1/1 -> Unit Delay/1, latched/1
  set/1 -> Switch1/1, Logical Operator/1
  reset/1 -> Switch2/2, Logical Operator1/1
  Unit Delay/1 -> Switch2/3
  Switch2/1 -> Switch1/3
  Logical Operator/1 -> Switch1/2
  Logical Operator1/1 -> Logical Operator/2, Switch2/1

== system ddm/DDM/DDM/TPM/LRPressureLow/SR_Latch1 ==
  set : Inport
  reset : Inport  Port=2
  Logical Operator : Logic  AllPortsSameDT=off  OutDataTypeStr=boolean
  Logical Operator1 : Logic  Operator=NOT  AllPortsSameDT=off  OutDataTypeStr=boolean
  Switch1 : Switch  Criteria=u2 ~= 0  Threshold=0.5
      settings: AttributesFormatString=<Criteria=%<Criteria>>
  Switch2 : Switch  Criteria=u2 ~= 0  Threshold=0.5
      settings: AttributesFormatString=<Criteria=%<Criteria>>
  Unit Delay : UnitDelay  SampleTime=-1  HasFrameUpgradeWarning=on
  latched : Outport
  wires:
  Switch1/1 -> Unit Delay/1, latched/1
  set/1 -> Switch1/1, Logical Operator/1
  reset/1 -> Switch2/2, Logical Operator1/1
  Unit Delay/1 -> Switch2/3
  Switch2/1 -> Switch1/3
  Logical Operator/1 -> Switch1/2
  Logical Operator1/1 -> Logical Operator/2, Switch2/1

== system ddm/DDM/DDM/TPM/LRSensorfail/SR_Latch1 ==
  set : Inport
  reset : Inport  Port=2
  Logical Operator : Logic  AllPortsSameDT=off  OutDataTypeStr=boolean
  Logical Operator1 : Logic  Operator=NOT  AllPortsSameDT=off  OutDataTypeStr=boolean
  Switch1 : Switch  Criteria=u2 ~= 0  Threshold=0.5
      settings: AttributesFormatString=<Criteria=%<Criteria>>
  Switch2 : Switch  Criteria=u2 ~= 0  Threshold=0.5
      settings: AttributesFormatString=<Criteria=%<Criteria>>
  Unit Delay : UnitDelay  SampleTime=-1  HasFrameUpgradeWarning=on
  latched : Outport
  wires:
  Switch1/1 -> Unit Delay/1, latched/1
  set/1 -> Switch1/1, Logical Operator/1
  reset/1 -> Switch2/2, Logical Operator1/1
  Unit Delay/1 -> Switch2/3
  Switch2/1 -> Switch1/3
  Logical Operator/1 -> Switch1/2
  Logical Operator1/1 -> Logical Operator/2, Switch2/1

== system ddm/DDM/DDM/TPM/LRWheelTmpHigh/SR_Latch1 ==
  set : Inport
  reset : Inport  Port=2
  Logical Operator : Logic  AllPortsSameDT=off  OutDataTypeStr=boolean
  Logical Operator1 : Logic  Operator=NOT  AllPortsSameDT=off  OutDataTypeStr=boolean
  Switch1 : Switch  Criteria=u2 ~= 0  Threshold=0.5
      settings: AttributesFormatString=<Criteria=%<Criteria>>
  Switch2 : Switch  Criteria=u2 ~= 0  Threshold=0.5
      settings: AttributesFormatString=<Criteria=%<Criteria>>
  Unit Delay : UnitDelay  SampleTime=-1  HasFrameUpgradeWarning=on
  latched : Outport
  wires:
  Switch1/1 -> Unit Delay/1, latched/1
  set/1 -> Switch1/1, Logical Operator/1
  reset/1 -> Switch2/2, Logical Operator1/1
  Unit Delay/1 -> Switch2/3
  Switch2/1 -> Switch1/3
  Logical Operator/1 -> Switch1/2
  Logical Operator1/1 -> Logical Operator/2, Switch2/1

== system ddm/DDM/DDM/TPM/RFBatwarn/SR_Latch1 ==
  set : Inport
  reset : Inport  Port=2
  Logical Operator : Logic  AllPortsSameDT=off  OutDataTypeStr=boolean
  Logical Operator1 : Logic  Operator=NOT  AllPortsSameDT=off  OutDataTypeStr=boolean
  Switch1 : Switch  Criteria=u2 ~= 0  Threshold=0.5
      settings: AttributesFormatString=<Criteria=%<Criteria>>
  Switch2 : Switch  Criteria=u2 ~= 0  Threshold=0.5
      settings: AttributesFormatString=<Criteria=%<Criteria>>
  Unit Delay : UnitDelay  SampleTime=-1  HasFrameUpgradeWarning=on
  latched : Outport
  wires:
  Switch1/1 -> Unit Delay/1, latched/1
  set/1 -> Switch1/1, Logical Operator/1
  reset/1 -> Switch2/2, Logical Operator1/1
  Unit Delay/1 -> Switch2/3
  Switch2/1 -> Switch1/3
  Logical Operator/1 -> Switch1/2
  Logical Operator1/1 -> Logical Operator/2, Switch2/1

== system ddm/DDM/DDM/TPM/RFPressureLow/SR_Latch1 ==
  set : Inport
  reset : Inport  Port=2
  Logical Operator : Logic  AllPortsSameDT=off  OutDataTypeStr=boolean
  Logical Operator1 : Logic  Operator=NOT  AllPortsSameDT=off  OutDataTypeStr=boolean
  Switch1 : Switch  Criteria=u2 ~= 0  Threshold=0.5
      settings: AttributesFormatString=<Criteria=%<Criteria>>
  Switch2 : Switch  Criteria=u2 ~= 0  Threshold=0.5
      settings: AttributesFormatString=<Criteria=%<Criteria>>
  Unit Delay : UnitDelay  SampleTime=-1  HasFrameUpgradeWarning=on
  latched : Outport
  wires:
  Switch1/1 -> Unit Delay/1, latched/1
  set/1 -> Switch1/1, Logical Operator/1
  reset/1 -> Switch2/2, Logical Operator1/1
  Unit Delay/1 -> Switch2/3
  Switch2/1 -> Switch1/3
  Logical Operator/1 -> Switch1/2
  Logical Operator1/1 -> Logical Operator/2, Switch2/1

== system ddm/DDM/DDM/TPM/RFSensorfail/SR_Latch1 ==
  set : Inport
  reset : Inport  Port=2
  Logical Operator : Logic  AllPortsSameDT=off  OutDataTypeStr=boolean
  Logical Operator1 : Logic  Operator=NOT  AllPortsSameDT=off  OutDataTypeStr=boolean
  Switch1 : Switch  Criteria=u2 ~= 0  Threshold=0.5
      settings: AttributesFormatString=<Criteria=%<Criteria>>
  Switch2 : Switch  Criteria=u2 ~= 0  Threshold=0.5
      settings: AttributesFormatString=<Criteria=%<Criteria>>
  Unit Delay : UnitDelay  SampleTime=-1  HasFrameUpgradeWarning=on
  latched : Outport
  wires:
  Switch1/1 -> Unit Delay/1, latched/1
  set/1 -> Switch1/1, Logical Operator/1
  reset/1 -> Switch2/2, Logical Operator1/1
  Unit Delay/1 -> Switch2/3
  Switch2/1 -> Switch1/3
  Logical Operator/1 -> Switch1/2
  Logical Operator1/1 -> Logical Operator/2, Switch2/1

== system ddm/DDM/DDM/TPM/RFWheelTmpHigh/SR_Latch1 ==
  set : Inport
  reset : Inport  Port=2
  Logical Operator : Logic  AllPortsSameDT=off  OutDataTypeStr=boolean
  Logical Operator1 : Logic  Operator=NOT  AllPortsSameDT=off  OutDataTypeStr=boolean
  Switch1 : Switch  Criteria=u2 ~= 0  Threshold=0.5
      settings: AttributesFormatString=<Criteria=%<Criteria>>
  Switch2 : Switch  Criteria=u2 ~= 0  Threshold=0.5
      settings: AttributesFormatString=<Criteria=%<Criteria>>
  Unit Delay : UnitDelay  SampleTime=-1  HasFrameUpgradeWarning=on
  latched : Outport
  wires:
  Switch1/1 -> Unit Delay/1, latched/1
  set/1 -> Switch1/1, Logical Operator/1
  reset/1 -> Switch2/2, Logical Operator1/1
  Unit Delay/1 -> Switch2/3
  Switch2/1 -> Switch1/3
  Logical Operator/1 -> Switch1/2
  Logical Operator1/1 -> Logical Operator/2, Switch2/1

== system ddm/DDM/DDM/TPM/RRBatwarn/SR_Latch1 ==
  set : Inport
  reset : Inport  Port=2
  Logical Operator : Logic  AllPortsSameDT=off  OutDataTypeStr=boolean
  Logical Operator1 : Logic  Operator=NOT  AllPortsSameDT=off  OutDataTypeStr=boolean
  Switch1 : Switch  Criteria=u2 ~= 0  Threshold=0.5
      settings: AttributesFormatString=<Criteria=%<Criteria>>
  Switch2 : Switch  Criteria=u2 ~= 0  Threshold=0.5
      settings: AttributesFormatString=<Criteria=%<Criteria>>
  Unit Delay : UnitDelay  SampleTime=-1  HasFrameUpgradeWarning=on
  latched : Outport
  wires:
  Switch1/1 -> Unit Delay/1, latched/1
  set/1 -> Switch1/1, Logical Operator/1
  reset/1 -> Switch2/2, Logical Operator1/1
  Unit Delay/1 -> Switch2/3
  Switch2/1 -> Switch1/3
  Logical Operator/1 -> Switch1/2
  Logical Operator1/1 -> Logical Operator/2, Switch2/1

== system ddm/DDM/DDM/TPM/RRPressureLow/SR_Latch1 ==
  set : Inport
  reset : Inport  Port=2
  Logical Operator : Logic  AllPortsSameDT=off  OutDataTypeStr=boolean
  Logical Operator1 : Logic  Operator=NOT  AllPortsSameDT=off  OutDataTypeStr=boolean
  Switch1 : Switch  Criteria=u2 ~= 0  Threshold=0.5
      settings: AttributesFormatString=<Criteria=%<Criteria>>
  Switch2 : Switch  Criteria=u2 ~= 0  Threshold=0.5
      settings: AttributesFormatString=<Criteria=%<Criteria>>
  Unit Delay : UnitDelay  SampleTime=-1  HasFrameUpgradeWarning=on
  latched : Outport
  wires:
  Switch1/1 -> Unit Delay/1, latched/1
  set/1 -> Switch1/1, Logical Operator/1
  reset/1 -> Switch2/2, Logical Operator1/1
  Unit Delay/1 -> Switch2/3
  Switch2/1 -> Switch1/3
  Logical Operator/1 -> Switch1/2
  Logical Operator1/1 -> Logical Operator/2, Switch2/1

== system ddm/DDM/DDM/TPM/RRSensorfail/SR_Latch1 ==
  set : Inport
  reset : Inport  Port=2
  Logical Operator : Logic  AllPortsSameDT=off  OutDataTypeStr=boolean
  Logical Operator1 : Logic  Operator=NOT  AllPortsSameDT=off  OutDataTypeStr=boolean
  Switch1 : Switch  Criteria=u2 ~= 0  Threshold=0.5
      settings: AttributesFormatString=<Criteria=%<Criteria>>
  Switch2 : Switch  Criteria=u2 ~= 0  Threshold=0.5
      settings: AttributesFormatString=<Criteria=%<Criteria>>
  Unit Delay : UnitDelay  SampleTime=-1  HasFrameUpgradeWarning=on
  latched : Outport
  wires:
  Switch1/1 -> Unit Delay/1, latched/1
  set/1 -> Switch1/1, Logical Operator/1
  reset/1 -> Switch2/2, Logical Operator1/1
  Unit Delay/1 -> Switch2/3
  Switch2/1 -> Switch1/3
  Logical Operator/1 -> Switch1/2
  Logical Operator1/1 -> Logical Operator/2, Switch2/1

== system ddm/DDM/DDM/TPM/RRWheelTmpHigh/SR_Latch1 ==
  set : Inport
  reset : Inport  Port=2
  Logical Operator : Logic  AllPortsSameDT=off  OutDataTypeStr=boolean
  Logical Operator1 : Logic  Operator=NOT  AllPortsSameDT=off  OutDataTypeStr=boolean
  Switch1 : Switch  Criteria=u2 ~= 0  Threshold=0.5
      settings: AttributesFormatString=<Criteria=%<Criteria>>
  Switch2 : Switch  Criteria=u2 ~= 0  Threshold=0.5
      settings: AttributesFormatString=<Criteria=%<Criteria>>
  Unit Delay : UnitDelay  SampleTime=-1  HasFrameUpgradeWarning=on
  latched : Outport
  wires:
  Switch1/1 -> Unit Delay/1, latched/1
  set/1 -> Switch1/1, Logical Operator/1
  reset/1 -> Switch2/2, Logical Operator1/1
  Unit Delay/1 -> Switch2/3
  Switch2/1 -> Switch1/3
  Logical Operator/1 -> Switch1/2
  Logical Operator1/1 -> Logical Operator/2, Switch2/1

== system ddm/DDM/DDM/VMC_DDM/ACC Acceleration Command Error/ACC Acceleration Command Error  ==
  note: Diagnostics and Fault Handling
  note: Release Condiction After Decision
  note: Test Pass Criteria
  note: Test Detection Criteria
  task_time_s : Inport
  VDDM_FCM1NoComCFS_flg : Inport  Port=2
  VDDM_FCM1RCErrCFS_flg : Inport  Port=3
  VDDM_FCM1CSErrCFS_flg : Inport  Port=4
  VVMC_ADASActive_flg : Inport  Port=5
  No_CAN6_BUS_OFF : Inport  Port=6
  VPMM_PowerSta_enum : Inport  Port=7
  VINP_ACCRequireAccel_mps2 : Inport  Port=8
  VINP_ADASACCSta_enum : Inport  Port=9
  DTC_clear_request : Inport  Port=10
  Abs : Abs
  Abs1 : Abs
  Constant1 : Constant  Value=KDDM_ACCAccelCmdErrDet_mps2
  Constant10 : Constant  Value=ENUM_ADASACCSTA_OFF
  Constant11 : Constant  Value=ENUM_ADASACCSTA_STANDBY
  Constant16 : Constant  Value=FALSE
  Constant2 : Constant  Value=FALSE
  Constant21 : Constant  Value=ZERO_INT
  Constant3 : Constant  Value=KDDM_ACCAccelCmdErrDet_mps2
  Constant30 : Constant  Value=ENUM_POWERSTA_OFF
  Constant31 : Constant  Value=ENUM_POWERSTA_STANDBY
  Constant32 : Constant  Value=TRUE
  Constant37 : Constant  Value=FALSE
  Constant38 : Constant  Value=KDDM_VMCDiagnosisOffSW_flg
  Constant4 : Constant  Value=KDDM_ACCAccelCmdErrDetTO_s
  Constant5 : Constant  Value=TRUE
  Constant6 : Constant  Value=KDDM_ACCAccelCmdErrPassTO_s
  Constant7 : Constant  Value=KDDM_ACCAccelCmdErrDTC_cnt
  Constant8 : Constant  Value=KDDM_ACCAccelCmdErrDTC_cnt
  Constant9 : Constant  Value=KDDM_ACCAccelCmdErrPassTO_s
  DTC_Couter1 : hcu_lib/Basic_Blocks/DTC_Couter
  DTC_Info : hcu_lib/Basic_Blocks/DTC_Info
  Equal1 : RelationalOperator  Operator=>  OutDataTypeStr=boolean  RndMeth=Simplest
  Equal{4..5,17..18} (4 alike) : RelationalOperator  Operator===  OutDataTypeStr=boolean  RndMeth=Simplest
  Equal2 : RelationalOperator  Operator=>  OutDataTypeStr=boolean  RndMeth=Simplest
  Equal3 : RelationalOperator  OutDataTypeStr=boolean  RndMeth=Simplest
  Logical Operator{1,4,6,11,17..18,20} (7 alike) : Logic  Operator=NOT  AllPortsSameDT=off  OutDataTypeStr=boolean
  Logical Operator10 : Logic  Inputs=5  AllPortsSameDT=off  OutDataTypeStr=boolean
  Logical Operator14 : Logic  AllPortsSameDT=off  OutDataTypeStr=boolean
  Logical Operator16 : Logic  Operator=OR  Inputs=4  AllPortsSameDT=off  OutDataTypeStr=boolean
  Logical Operator2 : Logic  Inputs=5  AllPortsSameDT=off  OutDataTypeStr=boolean
  Logical Operator3 : Logic  AllPortsSameDT=off  OutDataTypeStr=boolean
  Logical Operator5 : Logic  Operator=OR  AllPortsSameDT=off  OutDataTypeStr=boolean
  Relational Operator : RelationalOperator  Operator=>  OutDataTypeStr=boolean  RndMeth=Simplest
  Switch{2..3,5..6} (4 alike) : Switch  Criteria=u2 ~= 0
  Terminator : Terminator
  Test Detection Criteria : hcu_lib/Basic_Blocks/Test Detection Criteria
  Timer1 : hcu_lib/Basic_Blocks/Timer
  Unit Delay1 : UnitDelay  SampleTime=-1  HasFrameUpgradeWarning=on
  VDDM_ACCAccelCmdErrCFS_flg : Outport
  VDDM_ACCAccelCmdErrDetDTC_raw32 : Outport  Port=2
  wires:
  Constant11/1 -> Equal5/2
  Constant10/1 -> Equal4/1
  Logical Operator5/1 -> Logical Operator3/2
  Equal5/1 -> Logical Operator5/2
  Equal4/1 -> Logical Operator5/1
  [VINP_ADASACCSta_enum] -> Equal4/2, Equal5/1
  Logical Operator3/1 -> Logical Operator16/3
  Logical Operator14/1 -> Logical Operator16/1
  Unit Delay1/1 -> Equal17/1
  [VDDM_ACCAccelCmdErrPass_flg] -> Logical Operator3/1
  Constant8/1 -> DTC_Couter1/3
  Equal17/1 -> Logical Operator14/1
  Relational Operator/1 -> Terminator/1  "VDDM_ACCAccelCmdErrDFS_flg"
  Constant37/1 -> Switch6/3
  Logical Operator16/1 -> Switch6/2
  [VPMM_PowerSta_enum] -> Unit Delay1/1
  [VPMM_PowerSta_enum] -> Equal18/1
  Constant38/1 -> Logical Operator16/4
  [DTC_clear_request] -> Logical Operator16/2
  Constant30/1 -> Equal17/2
  DTC_Couter1/2 -> Relational Operator/1  "VDDM_ACCAccelCmdErrDTC_cnt"
  Constant32/1 -> Switch6/1
  Equal18/1 -> Logical Operator14/2
  Constant31/1 -> Equal18/2
  Constant21/1 -> Relational Operator/2
  DTC_Couter1/1 -> [VDDM_ACCAccelCmdErrCFS_flg]  "VDDM_ACCAccelCmdErrCFS_flg"
  Switch6/1 -> [VDDM_ACCAccelCmdErrCFSRls_flg]  "VDDM_ACCAccelCmdErrCFSRls_flg"
  [VDDM_ACCAccelCmdErrDet_flg] -> DTC_Couter1/1
  [VDDM_ACCAccelCmdErrCFSRls_flg] -> DTC_Couter1/2
  DTC_Info/1 -> VDDM_ACCAccelCmdErrDetDTC_raw32/1  "VDDM_ACCAccelCmdErrDetDTC_raw32"
  [DTC_clear_request] -> DTC_Info/4
  [VDDM_ACCAccelCmdErrCFS_flg] -> DTC_Info/3
  [VDDM_ACCAccelCmdErrPass_flg] -> DTC_Info/2
  [VDDM_ACCAccelCmdErrDet_flg] -> DTC_Info/1
  [VDDM_ACCAccelCmdErrCFSRls_flg] -> Switch5/2
  Constant16/1 -> Switch5/1
  Switch5/1 -> Test Detection Criteria/1
  VINP_ADASACCSta_enum/1 -> [VINP_ADASACCSta_enum]
  [VDDM_FCM1NoComCFS_flg] -> Logical Operator1/1
  Abs1/1 -> Equal1/1
  [No_CAN6_BUS_OFF] -> Logical Operator10/1
  [VDDM_FCM1CSErrCFS_flg] -> Logical Operator11/1
  Logical Operator10/1 -> Switch3/2
  Constant1/1 -> Equal1/2
  [VVMC_ADASActive_flg] -> Logical Operator10/5
  Equal1/1 -> Switch3/1
  Logical Operator4/1 -> Logical Operator10/3
  [VINP_ACCRequireAccel_mps2] -> Abs1/1
  Logical Operator11/1 -> Logical Operator10/4
  [VDDM_FCM1RCErrCFS_flg] -> Logical Operator4/1
  Logical Operator1/1 -> Logical Operator10/2
  Abs/1 -> Equal2/1
  VVMC_ADASActive_flg/1 -> [VVMC_ADASActive_flg]
  Equal2/1 -> Switch2/1
  Constant3/1 -> Equal2/2
  Constant9/1 -> Timer1/4
  [task_time_s] -> Timer1/3
  Test Detection Criteria/1 -> [VDDM_ACCAccelCmdErrDet_flg]  "VDDM_ACCAccelCmdErrDet_flg"
  Constant7/1 -> Test Detection Criteria/3
  Constant4/1 -> Test Detection Criteria/4
  [task_time_s] -> Test Detection Criteria/2
  task_time_s/1 -> [task_time_s]  "task_time_s"
  Switch3/1 -> Logical Operator6/1, Timer1/2
  Constant5/1 -> Switch3/3
  Logical Operator20/1 -> Logical Operator2/4
  Logical Operator18/1 -> Logical Operator2/3
  Logical Operator17/1 -> Logical Operator2/2
  [VINP_ACCRequireAccel_mps2] -> Abs/1
  [VDDM_FCM1CSErrCFS_flg] -> Logical Operator20/1
  [VDDM_FCM1RCErrCFS_flg] -> Logical Operator18/1
  [VDDM_FCM1NoComCFS_flg] -> Logical Operator17/1
  [VVMC_ADASActive_flg] -> Logical Operator2/5
  VINP_ACCRequireAccel_mps2/1 -> [VINP_ACCRequireAccel_mps2]
  No_CAN6_BUS_OFF/1 -> [No_CAN6_BUS_OFF]
  VDDM_FCM1CSErrCFS_flg/1 -> [VDDM_FCM1CSErrCFS_flg]
  VPMM_PowerSta_enum/1 -> [VPMM_PowerSta_enum]
  VDDM_FCM1RCErrCFS_flg/1 -> [VDDM_FCM1RCErrCFS_flg]
  DTC_clear_request/1 -> [DTC_clear_request]
  VDDM_FCM1NoComCFS_flg/1 -> [VDDM_FCM1NoComCFS_flg]
  Timer1/1 -> Equal3/1
  Constant2/1 -> Switch2/3
  Logical Operator6/1 -> Timer1/1
  Logical Operator2/1 -> Switch2/2
  [No_CAN6_BUS_OFF] -> Logical Operator2/1
  Constant6/1 -> Equal3/2
  [VDDM_ACCAccelCmdErrCFS_flg] -> VDDM_ACCAccelCmdErrCFS_flg/1
  Equal3/1 -> [VDDM_ACCAccelCmdErrPass_flg]  "VDDM_ACCAccelCmdErrPass_flg"
  Switch2/1 -> Switch5/3
